simulink model "Assignment"  (R2020b)
settings: Solver=FixedStepAuto  StartTime=0.0  StopTime=sim_time  FixedStep=0.001  RelTol=1e-3
undefined symbols (not defined in the file): A, b, B, C, D, i, J, Kb, Kt, L, r, R, W, X, Y, Z
libraries: simulink x4, simulink_extras x3
settings Model: Creator=Raana  LastModifiedBy=Raana
settings DataIOCC: ReturnWorkspaceOutputs=off

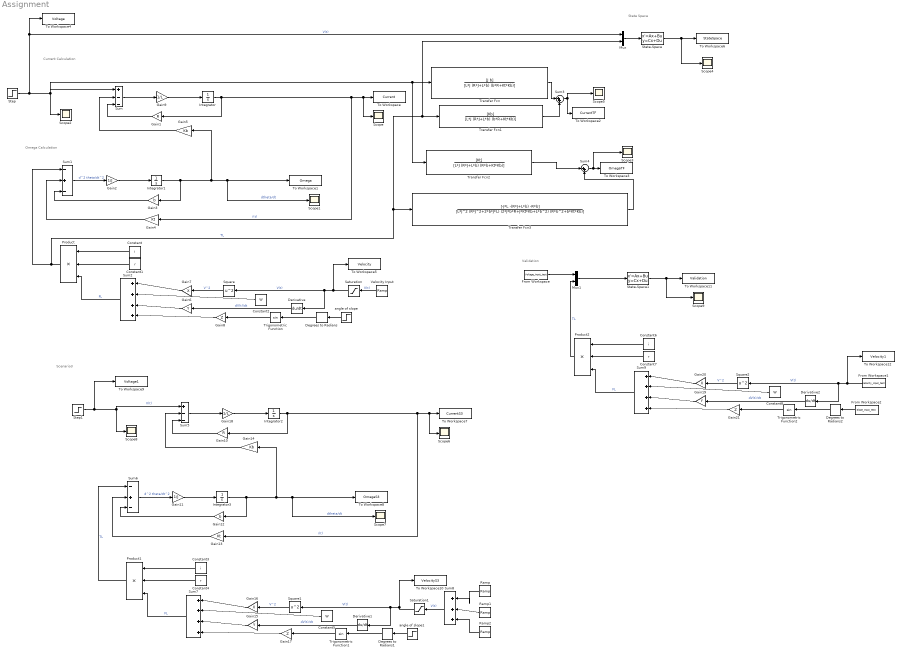
== system Assignment ==
  note: Validation
  note: Scenario3
  note: State Space
  note: Omega Calculation
  note: Current Calculation
  Constant : Constant  Value=i
  Constant1 : Constant  Value=r
  Constant2 : Constant  Value=W
  Constant3 : Constant  Value=i
  Constant4 : Constant  Value=r
  Constant5 : Constant  Value=W
  Constant6 : Constant  Value=i
  Constant7 : Constant  Value=r
  Constant8 : Constant  Value=W
  Degrees to Radians : simulink_extras/Transformations/Degrees to Radians
  Degrees to Radians1 : simulink_extras/Transformations/Degrees to Radians
  Degrees to Radians2 : simulink_extras/Transformations/Degrees to Radians
  Derivative : Derivative
  Derivative1 : Derivative
  Derivative2 : Derivative
  From Workspace : FromWorkspace  VariableName=Voltage_Input_test
  From Workspace1 : FromWorkspace  VariableName=Velocity_Input_test
  From Workspace2 : FromWorkspace  VariableName=Slope_Input_test
  Gain1 : Gain  Gain=R
  Gain10 : Gain  Gain=R
  Gain11 : Gain  Gain=1/J
  Gain12 : Gain  Gain=b
  Gain13 : Gain  Gain=Kt
  Gain14 : Gain  Gain=Kb
  Gain15 : Gain  Gain=Y
  Gain16 : Gain  Gain=X
  Gain17 : Gain  Gain=Z
  Gain18 : Gain  Gain=1/L
  Gain19 : Gain  Gain=Y
  Gain2 : Gain  Gain=1/J
  Gain20 : Gain  Gain=X
  Gain21 : Gain  Gain=Z
  Gain3 : Gain  Gain=b
  Gain4 : Gain  Gain=Kt
  Gain5 : Gain  Gain=Kb
  Gain6 : Gain  Gain=Y
  Gain7 : Gain  Gain=X
  Gain8 : Gain  Gain=Z
  Gain9 : Gain  Gain=1/L
  Integrator{,1..3} (4 alike) : Integrator
  Mux : Mux  Inputs=2
  Mux1 : Mux  Inputs=2
  Product : Product  Inputs=3
  Product1 : Product  Inputs=3
  Product2 : Product  Inputs=3
  Ramp : simulink/Sources/Ramp  slope=0.1  start=0.5  InitialOutput=0
  Ramp1 : simulink/Sources/Ramp  slope=0.12  start=20  InitialOutput=0
  Ramp2 : simulink/Sources/Ramp  slope=0.2  start=40  InitialOutput=0
  Saturation : Saturate  UpperLimit=10  LowerLimit=0
  Saturation1 : Saturate  UpperLimit=10
  Scope{,1..9} (10 alike) : Scope
  Square : Math  Operator=square  SaturateOnIntegerOverflow=on
  Square1 : Math  Operator=square  SaturateOnIntegerOverflow=on
  Square2 : Math  Operator=square  SaturateOnIntegerOverflow=on
  State-Space : StateSpace  A=A  B=B  C=C  D=D  InitialCondition=0
  State-Space1 : StateSpace  A=A  B=B  C=C  D=D  InitialCondition=0
  Step : Step  Time=0.1  After=48  SampleTime=0
  Step1 : Step  Time=0.1  After=48  SampleTime=0
  Sum : Sum  Inputs=|+--
  Sum1 : Sum  Inputs=|-+-
  Sum2 : Sum  Inputs=|++++
  Sum3 : Sum  Inputs=|++
  Sum4 : Sum  Inputs=|++
  Sum5 : Sum  Inputs=|+--
  Sum6 : Sum  Inputs=|-+-
  Sum7 : Sum  Inputs=|++++
  Sum8 : Sum  Inputs=|+++
  Sum9 : Sum  Inputs=|++++
  To Workspace : ToWorkspace  VariableName=Current  SampleTime=-1
  To Workspace1 : ToWorkspace  VariableName=Omega  SampleTime=-1
  To Workspace10 : ToWorkspace  VariableName=VelocityS3  SampleTime=-1
  To Workspace11 : ToWorkspace  VariableName=Validation  SampleTime=-1
  To Workspace12 : ToWorkspace  VariableName=Velocity1  SampleTime=-1
  To Workspace2 : ToWorkspace  VariableName=CurrentTF  SampleTime=-1
  To Workspace3 : ToWorkspace  VariableName=OmegaTF  SampleTime=-1
  To Workspace4 : ToWorkspace  VariableName=Voltage  SampleTime=-1
  To Workspace5 : ToWorkspace  VariableName=Velocity  SampleTime=-1
  To Workspace6 : ToWorkspace  VariableName=StateSpace  SampleTime=-1
  To Workspace7 : ToWorkspace  VariableName=CurrentS3  SampleTime=-1
  To Workspace8 : ToWorkspace  VariableName=OmegaS3  SampleTime=-1
  To Workspace9 : ToWorkspace  VariableName=Voltage1  SampleTime=-1
  Transfer Fcn : TransferFcn  Numerator=[J b]  Denominator=[L*J (R*J+L*b) (b*R+Kt*Kb)]
  Transfer Fcn1 : TransferFcn  Numerator=[Kb]  Denominator=[L*J (R*J+L*b) (b*R+Kt*Kb)]
  Transfer Fcn2 : TransferFcn  Numerator=[Kt]  Denominator=[L*J (R*J+L*b) (R*b+Kt*Kb)]
  Transfer Fcn3 : TransferFcn  Numerator=[-J*L -(R*J+L*b) -R*b]  Denominator=[L*J^2 (R*J^2+2*b*J*L) (2*J*b*R+J*Kt*Kb+L*b^2) (R*b^2+b*Kt*Kb)]
  Trigonometric Function : Trigonometry
  Trigonometric Function1 : Trigonometry
  Trigonometric Function2 : Trigonometry
  Velocity Input : simulink/Sources/Ramp  slope=1  start=0.5  InitialOutput=0
  angle of slope : Step  Time=0.5  After=3  SampleTime=0
  angle of slope1 : Step  Time=0.5  After=3  SampleTime=0
  wires:
  Step/1 -> To Workspace4/1, Mux/1, Sum/1, Transfer Fcn/1, Transfer Fcn2/1, Scope2/1  "V(t)"
  Integrator/1 -> Scope/1, To Workspace/1, Gain4/1, Gain1/1  "i(t)"
  Integrator1/1 -> Gain5/1, To Workspace1/1, Scope1/1, Gain3/1  "dtheta/dt"
  Gain3/1 -> Sum1/3
  Gain4/1 -> Sum1/2
  Gain1/1 -> Sum/3
  Gain5/1 -> Sum/2
  Product/1 -> Transfer Fcn3/1, Mux/2, Transfer Fcn1/1, Sum1/1  "TL"
  Square/1 -> Gain7/1  "V^2"
  Gain7/1 -> Sum2/1
  Constant2/1 -> Sum2/2
  Saturation/1 -> To Workspace5/1, Derivative/1, Square/1  "V(t)"
  Gain6/1 -> Sum2/3
  Gain8/1 -> Sum2/4
  Derivative/1 -> Gain6/1  "dV(t)/dt"
  Trigonometric Function/1 -> Gain8/1
  Constant/1 -> Product/1
  Constant1/1 -> Product/2
  Sum2/1 -> Product/3  "FL"
  angle of slope/1 -> Degrees to Radians/1
  Degrees to Radians/1 -> Trigonometric Function/1
  Transfer Fcn/1 -> Sum3/1
  Transfer Fcn1/1 -> Sum3/2
  Sum3/1 -> To Workspace2/1, Scope5/1
  Transfer Fcn2/1 -> Sum4/1
  Transfer Fcn3/1 -> Sum4/2
  Sum4/1 -> Scope3/1, To Workspace3/1
  Velocity Input/1 -> Saturation/1  "V(t)"
  State-Space/1 -> Scope4/1, To Workspace6/1
  Mux/1 -> State-Space/1
  Gain9/1 -> Integrator/1
  Sum/1 -> Gain9/1
  Gain2/1 -> Integrator1/1
  Sum1/1 -> Gain2/1  "d^2 theta/dt^2"
  Gain17/1 -> Sum7/4
  Gain11/1 -> Integrator3/1
  Degrees to Radians1/1 -> Trigonometric Function1/1
  Integrator3/1 -> Gain14/1, To Workspace8/1, Scope7/1, Gain12/1  "dtheta/dt"
  Sum5/1 -> Gain18/1
  Gain12/1 -> Sum6/3
  Gain13/1 -> Sum6/2
  Trigonometric Function1/1 -> Gain17/1
  Derivative1/1 -> Gain15/1  "dV(t)/dt"
  Constant3/1 -> Product1/1
  Constant4/1 -> Product1/2
  Square1/1 -> Gain16/1  "V^2"
  Gain15/1 -> Sum7/3
  Gain10/1 -> Sum5/3
  Gain14/1 -> Sum5/2
  Gain16/1 -> Sum7/1
  Integrator2/1 -> Scope6/1, To Workspace7/1, Gain13/1, Gain10/1  "i(t)"
  Step1/1 -> To Workspace9/1, Sum5/1, Scope8/1  "V(t)"
  Product1/1 -> Sum6/1  "TL"
  Sum6/1 -> Gain11/1  "d^2 theta/dt^2"
  Sum7/1 -> Product1/3  "FL"
  angle of slope1/1 -> Degrees to Radians1/1
  Constant5/1 -> Sum7/2
  Saturation1/1 -> To Workspace10/1, Derivative1/1, Square1/1  "V(t)"
  Gain18/1 -> Integrator2/1
  Ramp1/1 -> Sum8/2
  Ramp/1 -> Sum8/1
  Ramp2/1 -> Sum8/3
  Sum8/1 -> Saturation1/1  "V(t)"
  State-Space1/1 -> Scope9/1, To Workspace11/1
  Gain21/1 -> Sum9/4
  Sum9/1 -> Product2/3  "FL"
  Constant8/1 -> Sum9/2
  Square2/1 -> Gain20/1  "V^2"
  Gain19/1 -> Sum9/3
  From Workspace1/1 -> To Workspace12/1, Derivative2/1, Square2/1  "V(t)"
  Gain20/1 -> Sum9/1
  Degrees to Radians2/1 -> Trigonometric Function2/1
  Constant6/1 -> Product2/1
  Trigonometric Function2/1 -> Gain21/1
  Constant7/1 -> Product2/2
  Derivative2/1 -> Gain19/1  "dV(t)/dt"
  From Workspace2/1 -> Degrees to Radians2/1
  Product2/1 -> Mux1/2  "TL"
  Mux1/1 -> State-Space1/1
  From Workspace/1 -> Mux1/1
